simulink model "tab"  (R2024b)
settings: Solver=VariableStepAuto  StartTime=0.0  StopTime=0.5  RelTol=1e-3
InitFcn:
  | clc;
  | clear;
  | 
  | Vdc = 100;
  | 
  | R1 = 1e-3;
  | L1 = 4.1637e-6;
  | Lm = 0.0037;
  | 
  | R2 = 1e-3;
  | L2 = 7.6757e-4;
  | n2 = 0.4619;
  | 
  | R3 = 1e-3;
  | L3 = 7.6766e-4;
  | n3 = 0.4619;
libraries: spsSeriesRLCBranchLib x4, spsCurrentMeasurementLib x3, spsDCVoltageSourceLib x3, spsLinearTransformerLib x3, spsMeanLib x3, spsFullBridgeConverterLib x3, spsGroundLib x1, spspowerguiLib x1
settings Model: Creator=wang.shum  LastModifiedBy=marco

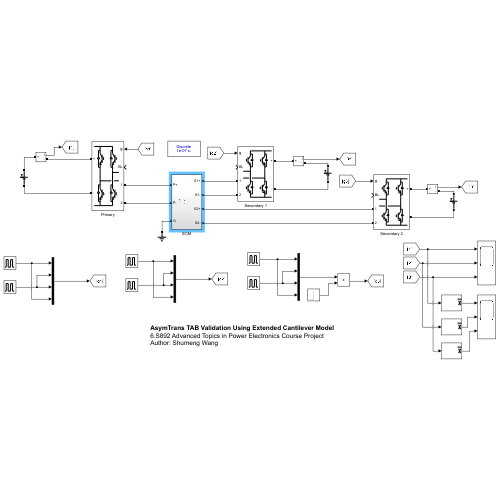
[thumbnail: Simulink's stored preview of the top-level diagram]
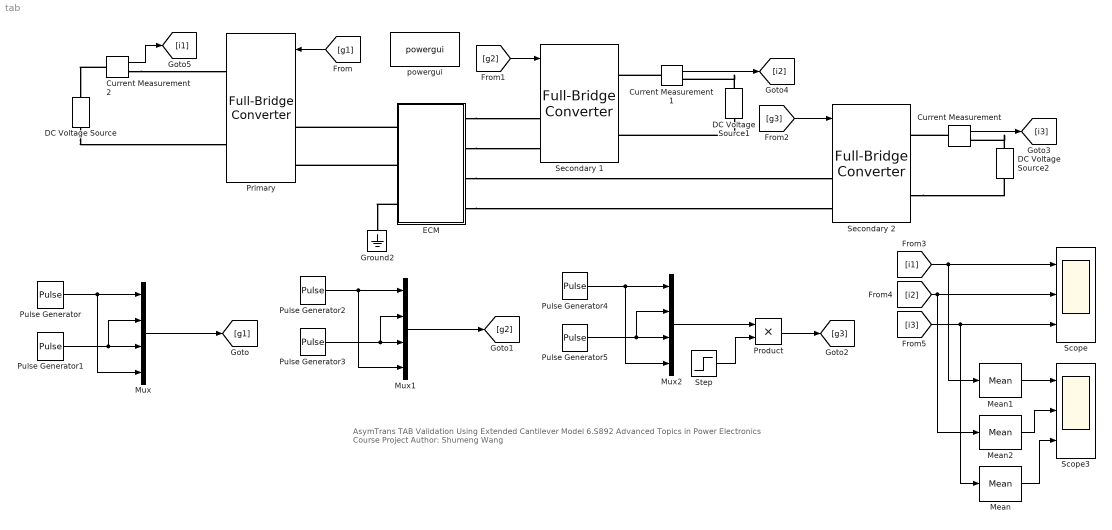
== system tab ==
  note: AsymTrans TAB Validation Using Extended Cantilever Model
      | 6.S892 Advanced Topics in Power Electronics Course Project
      | Author: Shumeng Wang
  Current Measurement : spsCurrentMeasurementLib/Current Measurement  PhasorSimulation=off  OutputType=Complex  PSBequivalent=0
  Current Measurement1 : spsCurrentMeasurementLib/Current Measurement  PhasorSimulation=off  OutputType=Complex  PSBequivalent=0
  Current Measurement2 : spsCurrentMeasurementLib/Current Measurement  PhasorSimulation=off  OutputType=Complex  PSBequivalent=0
  DC Voltage Source : spsDCVoltageSourceLib/DC Voltage Source  Amplitude=Vdc  Measurements=None
  DC Voltage Source1 : spsDCVoltageSourceLib/DC Voltage Source  Amplitude=Vdc  Measurements=None
  DC Voltage Source2 : spsDCVoltageSourceLib/DC Voltage Source  Amplitude=Vdc  Measurements=None
  ECM : Subsystem
  Ground2 : spsGroundLib/Ground  LConnTagsString=a
  Mean : spsMeanLib/Mean  Freq=1e5  Vinit=0  Ts=0
  Mean1 : spsMeanLib/Mean  Freq=1e5  Vinit=0  Ts=0
  Mean2 : spsMeanLib/Mean  Freq=1e5  Vinit=0  Ts=0
  Mux : Mux
  Mux1 : Mux
  Mux2 : Mux
  Primary : spsFullBridgeConverterLib/Full-Bridge Converter  ModelType=Switching devices  Ron=1e-3  Rs=1e6  Cs=inf  Vforward=[0,0]  Ron_Diode=1e-3  Rs_Diode=1e6  Cs_Diode=inf  Vf_Diode=1e-3  Rs_CurrentSource=inf  Ron_ACsource=1e-3
      settings: LibrarySourceBlock=sps_lib/Power Electronics/Full-Bridge Converter
  Product : Product
  Pulse Generator : DiscretePulseGenerator  PulseType=Time based  Period=1e-5  PulseWidth=50
  Pulse Generator1 : DiscretePulseGenerator  PulseType=Time based  Period=1e-5  PulseWidth=50  PhaseDelay=0.5e-5
  Pulse Generator2 : DiscretePulseGenerator  PulseType=Time based  Period=1e-5  PulseWidth=50  PhaseDelay=0.2e-5
  Pulse Generator3 : DiscretePulseGenerator  PulseType=Time based  Period=1e-5  PulseWidth=50  PhaseDelay=0.7e-5
  Pulse Generator4 : DiscretePulseGenerator  PulseType=Time based  Period=1e-5  PulseWidth=50  PhaseDelay=0.1e-5
  Pulse Generator5 : DiscretePulseGenerator  PulseType=Time based  Period=1e-5  PulseWidth=50  PhaseDelay=0.6e-5
  Scope : Scope  NumInputPorts=3
  Scope3 : Scope  NumInputPorts=3
  Secondary 1 : spsFullBridgeConverterLib/Full-Bridge Converter  ModelType=Switching devices  Ron=1e-3  Rs=1e6  Cs=inf  Vforward=[0,0]  Ron_Diode=1e-3  Rs_Diode=1e6  Cs_Diode=inf  Vf_Diode=1e-3  Rs_CurrentSource=inf  Ron_ACsource=1e-3
      settings: LibrarySourceBlock=sps_lib/Power Electronics/Full-Bridge Converter
  Secondary 2 : spsFullBridgeConverterLib/Full-Bridge Converter  ModelType=Switching devices  Ron=1e-3  Rs=1e6  Cs=inf  Vforward=[0,0]  Ron_Diode=1e-3  Rs_Diode=1e6  Cs_Diode=inf  Vf_Diode=1e-3  Rs_CurrentSource=inf  Ron_ACsource=1e-3
      settings: LibrarySourceBlock=sps_lib/Power Electronics/Full-Bridge Converter
  Step : Step  Time=0.3  SampleTime=0
  powergui : spspowerguiLib/powergui  Priority=1  SimulationMode=Discrete  SampleTime=1e-7  frequency=60  Iterations=50  frequencyindice=0  Pbase=100e6  ErrMax=1e-4  UnitsV=kV  UnitsW=MW  buscounter=0  FunctionMessages=off  echomessages=off  EnableUseOfTLC=off  CurrentSourceSwitches=off  DisableSnubberDevices=off  DisableRonSwitches=off  DisableVfSwitches=off  DisplayEquations=off  AutomaticDiscreteSolvers=off  SolverType=Tustin/Backward Euler (TBE)  Interpol=off  ExternalGateDelay=off  methode=off  Ts=100  x0status=blocks  SPID=on  SwTol=0  HookPort=off  NonlinearTolerance=1e-4  nMaxIteration=100  ContinueOnMaxIteration=off  RestoreLinks=warning  ResistiveCurrentMeasurement=off  Frange=[0:2:500]  Ylog=off  Xlog=on  ShowGrid=off  save=off  variable=ZData  structure=0  ZoomFFT=off  StartTime=0.0  cycles=1  DisplayStyle=1  fundamental=60  FreqAxis=off  MaxFrequency=1000  frequencyindicesteady=1  RmsSteady=1  display=off
  wires:
  Pulse Generator/1 -> Mux/4, Mux/1
  Pulse Generator1/1 -> Mux/2, Mux/3
  Mux/1 -> [g1]
  [g1] -> Primary/1
  Mux1/1 -> [g2]
  Pulse Generator4/1 -> Mux2/4, Mux2/1
  Pulse Generator5/1 -> Mux2/2, Mux2/3
  [g2] -> Secondary 1/1
  [g3] -> Secondary 2/1
  Current Measurement/1 -> [i3]
  Current Measurement1/1 -> [i2]
  Current Measurement2/1 -> [i1]
  [i1] -> Mean1/1, Scope/1
  [i2] -> Mean2/1, Scope/2
  [i3] -> Mean/1, Scope/3
  Pulse Generator2/1 -> Mux1/4, Mux1/1
  Pulse Generator3/1 -> Mux1/3, Mux1/2
  Mux2/1 -> Product/1
  Product/1 -> [g3]
  Step/1 -> Product/2
  Mean1/1 -> Scope3/1
  Mean2/1 -> Scope3/2
  Mean/1 -> Scope3/3
  connections:
  ECM/LConn2 -- Primary/LConn2
  ECM/LConn1 -- Primary/LConn1
  ECM/RConn2 -- Secondary 1/LConn2
  ECM/RConn1 -- Secondary 1/LConn1
  ECM/RConn3 -- Secondary 2/LConn1
  ECM/RConn4 -- Secondary 2/LConn2
  DC Voltage Source/LConn1 -- Primary/RConn2
  DC Voltage Source1/LConn1 -- Secondary 1/RConn2
  Secondary 2/RConn2 -- DC Voltage Source2/LConn1
  Current Measurement/LConn1 -- Secondary 2/RConn1
  DC Voltage Source2/RConn1 -- Current Measurement/RConn1
  Current Measurement1/LConn1 -- Secondary 1/RConn1
  DC Voltage Source1/RConn1 -- Current Measurement1/RConn1
  Current Measurement2/RConn1 -- Primary/RConn1
  Current Measurement2/LConn1 -- DC Voltage Source/RConn1
  ECM/LConn3 -- Ground2/LConn1

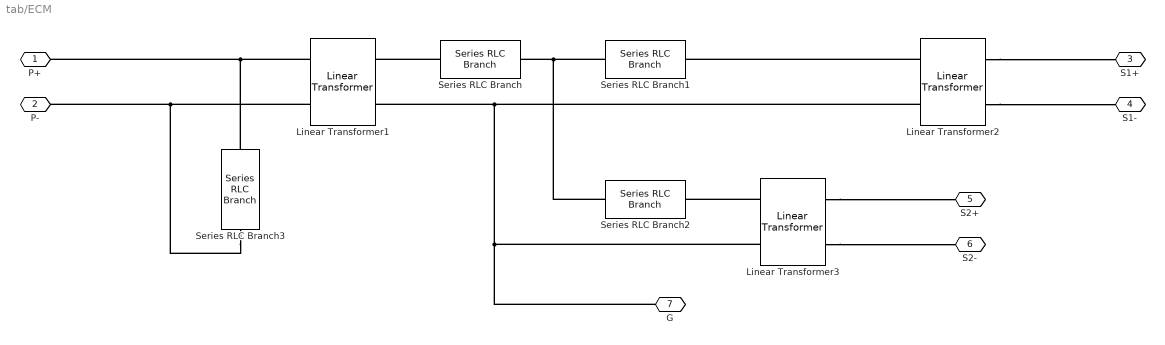
== system tab/ECM ==
  Linear Transformer1 : spsLinearTransformerLib/Linear Transformer  UNITS=SI  NominalPower=[1e3 1e5 ]  winding1=[100 1e-3 1e-9]  winding2=[100 1e-3 1e-9]  ThreeWindings=off  winding3=[3.15e+05 1.9845e+05 12.634]  RmLm=[5000 5]  Measurements=None  DataType=on
  Linear Transformer2 : spsLinearTransformerLib/Linear Transformer  UNITS=SI  NominalPower=[1e3 1e5 ]  winding1=[100 1e-3 1e-9]  winding2=[100*n2 1e-3 1e-9]  ThreeWindings=off  winding3=[3.15e+05 1.9845e+05 12.634]  RmLm=[5000 5]  Measurements=None  DataType=on
  Linear Transformer3 : spsLinearTransformerLib/Linear Transformer  UNITS=SI  NominalPower=[1e3 1e5 ]  winding1=[100 1e-3 1e-9]  winding2=[100*n3 1e-3 1e-9]  ThreeWindings=off  winding3=[3.15e+05 1.9845e+05 12.634]  RmLm=[5000 5]  Measurements=None  DataType=on
  Series RLC Branch : spsSeriesRLCBranchLib/Series RLC Branch  LConnTagsString=__new0  RConnTagsString=__new0  BranchType=RL  Resistance=R1  Inductance=L1  SetiL0=off  InitialCurrent=0  Capacitance=1e-6  Setx0=off  InitialVoltage=0  Measurements=None
  Series RLC Branch1 : spsSeriesRLCBranchLib/Series RLC Branch  LConnTagsString=__new0  RConnTagsString=__new0  BranchType=RL  Resistance=R2  Inductance=L2  SetiL0=off  InitialCurrent=0  Capacitance=1e-6  Setx0=off  InitialVoltage=0  Measurements=None
  Series RLC Branch2 : spsSeriesRLCBranchLib/Series RLC Branch  LConnTagsString=__new0  RConnTagsString=__new0  BranchType=RL  Resistance=R3  Inductance=L3  SetiL0=off  InitialCurrent=0  Capacitance=1e-6  Setx0=off  InitialVoltage=0  Measurements=None
  Series RLC Branch3 : spsSeriesRLCBranchLib/Series RLC Branch  LConnTagsString=__new0  RConnTagsString=__new0  BranchType=RL  Resistance=R1  Inductance=Lm  SetiL0=off  InitialCurrent=0  Capacitance=1e-6  Setx0=off  InitialVoltage=0  Measurements=None
  P+ : PMIOPort  Side=Left
  P- : PMIOPort  Port=2  Side=Left
  S1+ : PMIOPort  Port=3  Side=Right
  S1- : PMIOPort  Port=4  Side=Right
  S2+ : PMIOPort  Port=5  Side=Right
  S2- : PMIOPort  Port=6  Side=Right
  G : PMIOPort  Port=7  Side=Left
  connections:
  Linear Transformer2/LConn1 -- Series RLC Branch1/RConn1
  Linear Transformer2/LConn2 -- Linear Transformer1/RConn2 -- Linear Transformer3/LConn2 -- G/RConn1
  Linear Transformer3/RConn2 -- S2-/RConn1
  Linear Transformer3/RConn1 -- S2+/RConn1
  Linear Transformer3/LConn1 -- Series RLC Branch2/RConn1
  Series RLC Branch2/LConn1 -- Series RLC Branch1/LConn1 -- Series RLC Branch/RConn1
  Series RLC Branch/LConn1 -- Linear Transformer1/RConn1
  Series RLC Branch3/RConn1 -- Linear Transformer1/LConn2 -- P-/RConn1
  P+/RConn1 -- Linear Transformer1/LConn1 -- Series RLC Branch3/LConn1
  Linear Transformer2/RConn2 -- S1-/RConn1
  Linear Transformer2/RConn1 -- S1+/RConn1
